simulink model "satellite_control_magnetorquer_model"  (R2017a)
settings: Solver=ode3  StartTime=0.0  StopTime=1000  FixedStep=dt  RelTol=1e-3  EnableMultiTasking=on
undefined symbols (not defined in the file or in its folder): imu_sigma, q_0, w_B_IB_0, w_O
settings Model: Creator=Goh  LastModifiedBy=Rusty Goh
settings DataIOCC: SaveFormat=Array
settings OptimizationCC: LifeSpan=inf
settings DebuggingCC: UnderspecifiedInitializationDetection=Classic  MergeDetectMultiDrivingBlocksExec=none  StateNameClashWarn=warning  SFUnexpectedBacktrackingDiag=warning  SFNoUnconditionalDefaultTransitionDiag=warning  SFExecutionAtInitializationDiag=none
settings HardwareCC: ProdBitPerPointer=32  ProdBitPerSizeT=32  ProdBitPerPtrDiffT=32  ProdLargestAtomicFloat=None  ProdIntDivRoundTo=Undefined  ProdEndianess=Unspecified  ProdWordSize=32  ProdHWDeviceType=32-bit Generic
settings ModelReferenceCC: PropagateSignalLabelsOutOfModel=off
settings GRTTargetCC: TargetLangStandard=C89/C90 (ANSI)  GeneratePreprocessorConditionals=Disable all
settings ConfigComp: CovMetricSettings=dw  CovHtmlReporting=on  CovSaveCumulativeToWorkspaceVar=on  CovSaveSingleToWorkspaceVar=on  CovExternalEMLEnable=off

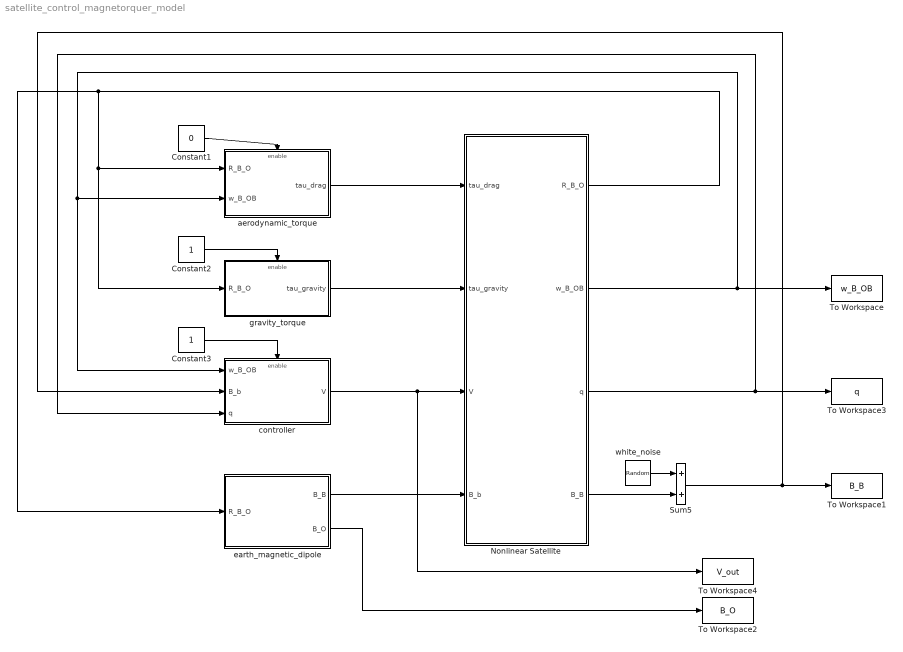
== system satellite_control_magnetorquer_model ==
  Constant1 : Constant  Value=0
  Constant2 : Constant
  Constant3 : Constant
  "Nonlinear Satellite " : Subsystem
  Sum5 : Sum  SaturateOnIntegerOverflow=on
  To Workspace : ToWorkspace  VariableName=w_B_OB  SampleTime=-1
  To Workspace1 : ToWorkspace  VariableName=B_B  SampleTime=-1
  To Workspace2 : ToWorkspace  VariableName=B_O  SampleTime=-1
  To Workspace3 : ToWorkspace  VariableName=q  SampleTime=-1
  To Workspace4 : ToWorkspace  VariableName=V_out  SampleTime=-1
  aerodynamic_torque : Subsystem
  controller : Subsystem
  earth_magnetic_dipole : Subsystem
  gravity_torque : Subsystem
  white_noise : RandomNumber  Variance=imu_sigma^2  SampleTime=0
  wires:
  "Nonlinear Satellite "/2(w_B_OB) -> To Workspace/1, controller/1(w_B_OB), aerodynamic_torque/2(w_B_OB)
  "Nonlinear Satellite "/3(q) -> controller/3(q), To Workspace3/1
  gravity_torque/1(tau_gravity) -> "Nonlinear Satellite "/2(tau_gravity)
  "Nonlinear Satellite "/1(R_B_O) -> gravity_torque/1(R_B_O), aerodynamic_torque/1(R_B_O), earth_magnetic_dipole/1(R_B_O)
  aerodynamic_torque/1(tau_drag) -> "Nonlinear Satellite "/1(tau_drag)
  earth_magnetic_dipole/1(B_B) -> "Nonlinear Satellite "/4(B_b)
  earth_magnetic_dipole/2(B_O) -> To Workspace2/1
  Constant1/1 -> aerodynamic_torque/Enable
  Constant2/1 -> gravity_torque/Enable
  Constant3/1 -> controller/Enable
  controller/1(V) -> "Nonlinear Satellite "/3(V), To Workspace4/1
  white_noise/1 -> Sum5/1
  "Nonlinear Satellite "/4(B_B) -> Sum5/2
  Sum5/1 -> controller/2(B_b), To Workspace1/1

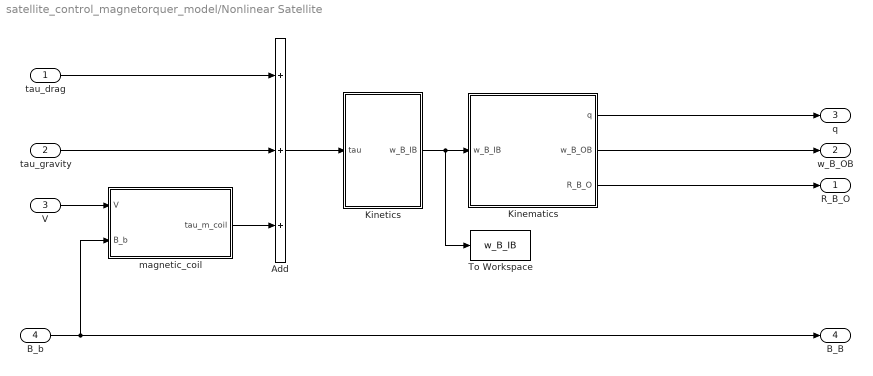
== system satellite_control_magnetorquer_model/Nonlinear Satellite  ==
  tau_drag : Inport
  tau_gravity : Inport  Port=2
  V : Inport  Port=3
  B_b : Inport  Port=4
  Add : Sum  Inputs=+++
  Kinematics : Subsystem
  Kinetics : Subsystem
  To Workspace : ToWorkspace  VariableName=w_B_IB  SampleTime=-1
  "magnetic_coil " : Subsystem
  R_B_O : Outport
  w_B_OB : Outport  Port=2
  q : Outport  Port=3
  B_B : Outport  Port=4
  wires:
  Kinematics/2(w_B_OB) -> w_B_OB/1
  Kinematics/1(q) -> q/1
  Kinematics/3(R_B_O) -> R_B_O/1
  Kinetics/1(w_B_IB) -> Kinematics/1(w_B_IB), To Workspace/1
  Add/1 -> Kinetics/1(tau)
  tau_drag/1 -> Add/1
  tau_gravity/1 -> Add/2
  V/1 -> "magnetic_coil "/1(V)
  B_b/1 -> B_B/1, "magnetic_coil "/2(B_b)
  "magnetic_coil "/1(tau_m_coil) -> Add/3

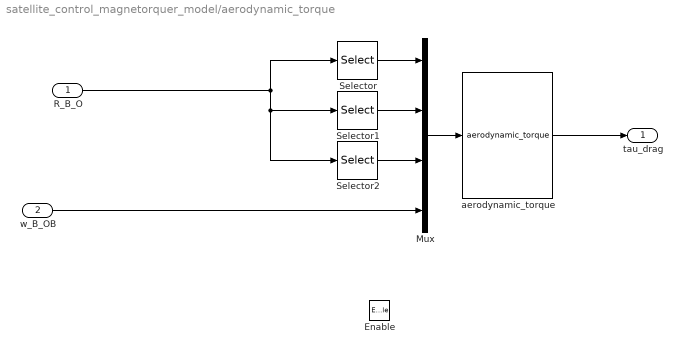
== system satellite_control_magnetorquer_model/aerodynamic_torque ==
  R_B_O : Inport
  w_B_OB : Inport  Port=2
  Enable : EnablePort
  Mux : Mux
  Selector : Selector  NumberOfDimensions=2  InputPortWidth=3  IndexOptions=Index vector (dialog),Index vector (dialog)  Indices=[1:3],1  OutputSizes=1,1
  Selector1 : Selector  NumberOfDimensions=2  InputPortWidth=3  IndexOptions=Index vector (dialog),Index vector (dialog)  Indices=[1:3],2  OutputSizes=1,1
  Selector2 : Selector  NumberOfDimensions=2  InputPortWidth=3  IndexOptions=Index vector (dialog),Index vector (dialog)  Indices=[1:3],3  OutputSizes=1,1
  aerodynamic_torque : MATLABFcn  MATLABFcn=aerodynamic_torque  OutputDimensions=[3,1]  Output1D=off
  tau_drag : Outport
  wires:
  R_B_O/1 -> Selector2/1, Selector1/1, Selector/1
  w_B_OB/1 -> Mux/4
  aerodynamic_torque/1 -> tau_drag/1
  Mux/1 -> aerodynamic_torque/1
  Selector2/1 -> Mux/3
  Selector/1 -> Mux/1
  Selector1/1 -> Mux/2

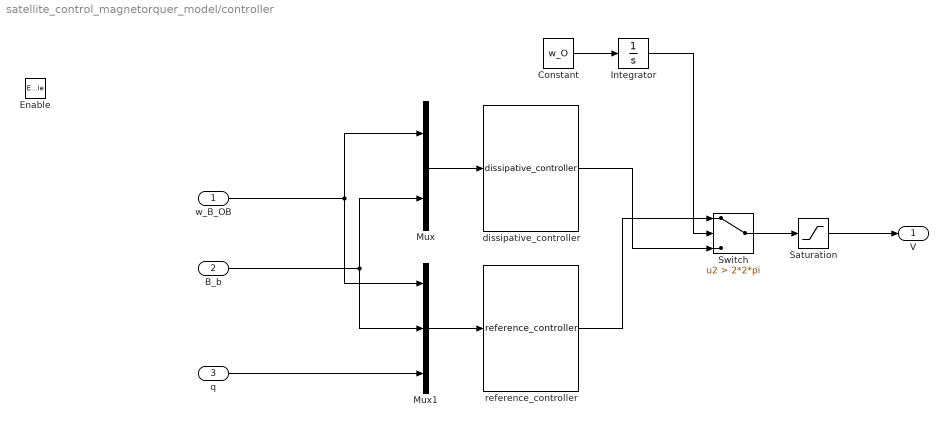
== system satellite_control_magnetorquer_model/controller ==
  w_B_OB : Inport
  B_b : Inport  Port=2
  q : Inport  Port=3
  Enable : EnablePort
  Constant : Constant  Value=w_O
  Integrator : Integrator
  Mux : Mux  Inputs=2
  Mux1 : Mux  Inputs=3
  Saturation : Saturate  UpperLimit=5  LowerLimit=-5
  Switch : Switch  Criteria=u2 > Threshold  Threshold=2*2*pi
  dissipative_controller : MATLABFcn  MATLABFcn=dissipative_controller  OutputDimensions=[3,1]  Output1D=off
  reference_controller : MATLABFcn  MATLABFcn=reference_controller  OutputDimensions=[3,1]  Output1D=off
  V : Outport
  wires:
  w_B_OB/1 -> Mux/1, Mux1/1
  B_b/1 -> Mux/2, Mux1/2
  Mux/1 -> dissipative_controller/1
  reference_controller/1 -> Switch/1
  Mux1/1 -> reference_controller/1
  q/1 -> Mux1/3
  dissipative_controller/1 -> Switch/3
  Integrator/1 -> Switch/2
  Constant/1 -> Integrator/1
  Switch/1 -> Saturation/1
  Saturation/1 -> V/1

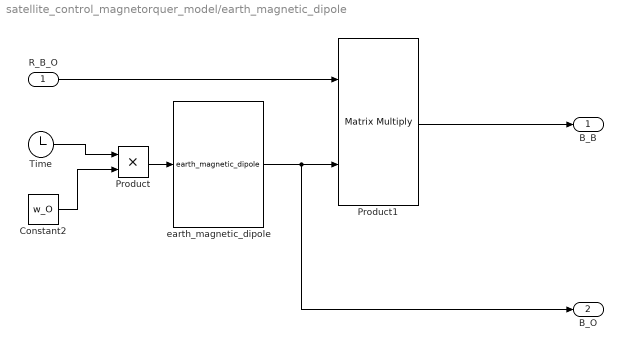
== system satellite_control_magnetorquer_model/earth_magnetic_dipole ==
  R_B_O : Inport
  Constant2 : Constant  Value=w_O  VectorParams1D=off
  Product : Product
  Product1 : Product  Multiplication=Matrix(*)
  Time : Clock
  earth_magnetic_dipole : MATLABFcn  MATLABFcn=earth_magnetic_dipole  OutputDimensions=[3,1]  Output1D=off
  B_B : Outport
  B_O : Outport  Port=2
  wires:
  earth_magnetic_dipole/1 -> B_O/1, Product1/2
  R_B_O/1 -> Product1/1
  Time/1 -> Product/1
  Constant2/1 -> Product/2
  Product/1 -> earth_magnetic_dipole/1
  Product1/1 -> B_B/1

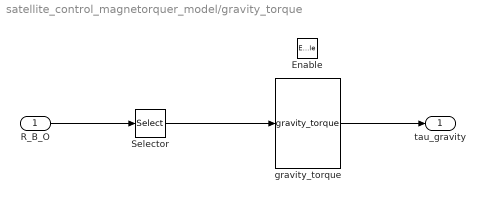
== system satellite_control_magnetorquer_model/gravity_torque ==
  R_B_O : Inport
  Enable : EnablePort
  Selector : Selector  NumberOfDimensions=2  InputPortWidth=3  IndexOptions=Index vector (dialog),Index vector (dialog)  Indices=[1:3],[3]  OutputSizes=1,1
  gravity_torque : MATLABFcn  MATLABFcn=gravity_torque  OutputDimensions=[3,1]  Output1D=off
  tau_gravity : Outport
  wires:
  gravity_torque/1 -> tau_gravity/1
  Selector/1 -> gravity_torque/1
  R_B_O/1 -> Selector/1

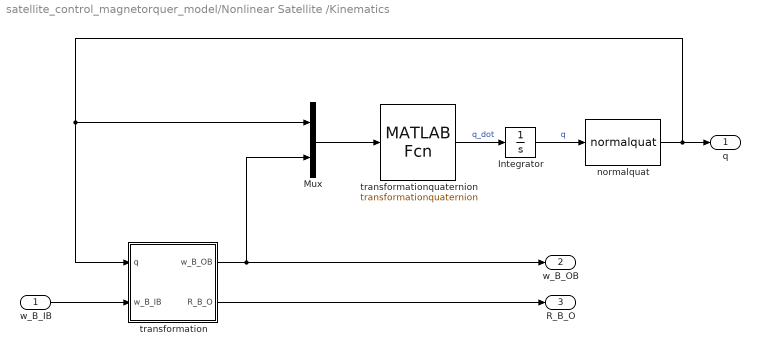
== system satellite_control_magnetorquer_model/Nonlinear Satellite /Kinematics ==
  w_B_IB : Inport
  Integrator : Integrator  InitialCondition=q_0
  Mux : Mux  Inputs=2
  normalquat : MATLABFcn  MATLABFcn=normalquat  OutputDimensions=[4,1]  Output1D=off
  transformation : Subsystem
  transformationquaternion : MATLABFcn  MATLABFcn=transformationquaternion  OutputDimensions=[4,1]  Output1D=off
  q : Outport
  w_B_OB : Outport  Port=2
  R_B_O : Outport  Port=3
  wires:
  Integrator/1 -> normalquat/1  "q"
  transformationquaternion/1 -> Integrator/1  "q_dot"
  w_B_IB/1 -> transformation/2(w_B_IB)
  transformation/1(w_B_OB) -> Mux/2, w_B_OB/1
  transformation/2(R_B_O) -> R_B_O/1
  Mux/1 -> transformationquaternion/1
  normalquat/1 -> transformation/1(q), Mux/1, q/1

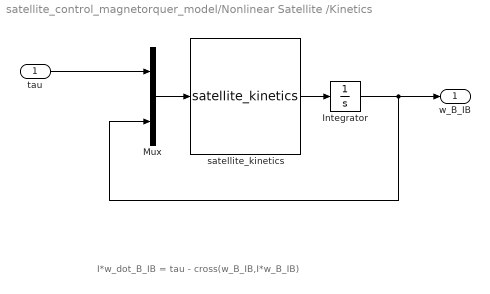
== system satellite_control_magnetorquer_model/Nonlinear Satellite /Kinetics ==
  note: I*w_dot_B_IB = tau - cross(w_B_IB,I*w_B_IB)
  tau : Inport
  Integrator : Integrator  InitialCondition=w_B_IB_0
  Mux : Mux  Inputs=[3 3]
  satellite_kinetics : MATLABFcn  MATLABFcn=satellite_kinetics  OutputDimensions=[3,1]  Output1D=off
  w_B_IB : Outport
  wires:
  Integrator/1 -> w_B_IB/1, Mux/2
  tau/1 -> Mux/1
  satellite_kinetics/1 -> Integrator/1
  Mux/1 -> satellite_kinetics/1

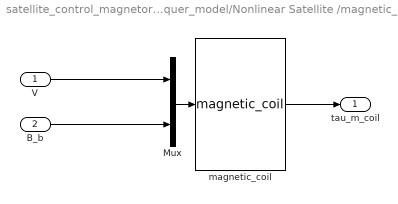
== system satellite_control_magnetorquer_model/Nonlinear Satellite /magnetic_coil  ==
  V : Inport
  B_b : Inport  Port=2
  Mux : Mux  Inputs=2
  magnetic_coil : MATLABFcn  MATLABFcn=magnetic_coil  OutputDimensions=[3,1]  Output1D=off
  tau_m_coil : Outport
  wires:
  V/1 -> Mux/1
  Mux/1 -> magnetic_coil/1
  magnetic_coil/1 -> tau_m_coil/1
  B_b/1 -> Mux/2

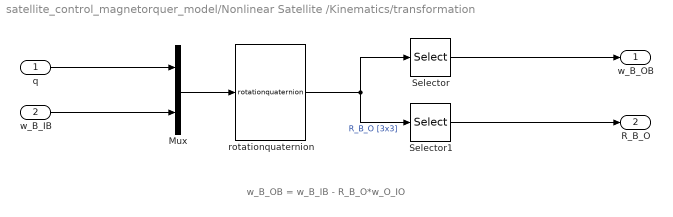
== system satellite_control_magnetorquer_model/Nonlinear Satellite /Kinematics/transformation ==
  note: w_B_OB = w_B_IB - R_B_O*w_O_IO
  q : Inport
  w_B_IB : Inport  Port=2
  Mux : Mux  Inputs=2
  Selector : Selector  NumberOfDimensions=2  InputPortWidth=3  IndexOptions=Index vector (dialog),Index vector (dialog)  Indices=[1:3],4  OutputSizes=1,1
  Selector1 : Selector  NumberOfDimensions=2  InputPortWidth=3  IndexOptions=Index vector (dialog),Index vector (dialog)  Indices=[1:3],[1:3]  OutputSizes=1,1
  rotationquaternion : MATLABFcn  MATLABFcn=rotationquaternion  OutputDimensions=[3,4]  Output1D=off
  w_B_OB : Outport
  R_B_O : Outport  Port=2
  wires:
  q/1 -> Mux/1
  Mux/1 -> rotationquaternion/1
  w_B_IB/1 -> Mux/2
  rotationquaternion/1 -> Selector/1, Selector1/1  "R_B_O [3x3]"
  Selector/1 -> w_B_OB/1
  Selector1/1 -> R_B_O/1
